simulink model "BMSOut"  (R2024a)
settings: Solver=FixedStepDiscrete  StartTime=0.0  StopTime=10000  RelTol=1e-3
undefined symbols (not defined in the file): PlntBattNumCellSer
settings Model: DataDictionary=VirtualVehicleTemplate.sldd  ModifiedByFormat=The MathWorks, Inc.  ExtModeTrigDuration=5  Creator=The MathWorks, Inc.  LastModifiedBy=The MathWorks, Inc.
settings SolverCC: AlgebraicLoopSolver=TrustRegion  PositivePriorityOrder=on  AutoInsertRateTranBlk=on  MaxZcPerStep=1
settings DataIOCC: ExternalInput=Battery  SaveOutput=off  SaveTime=off  SignalLoggingName=logsOut
settings OptimizationCC: BlockReduction=off  DefaultParameterBehavior=Inlined  UseFloatMulNetSlope=on  DefaultUnderspecifiedDataType=single  OptimizeBlockIOStorage=off  EnhancedBackFolding=on  PassReuseOutputArgsThreshold=0  ZeroExternalMemoryAtStartup=off  ZeroInternalMemoryAtStartup=off  EfficientFloat2IntCast=on  MaxStackSize=64  OptimizeBlockOrder=speed  DifferentSizesBufferReuse=on
settings DebuggingCC: SignalInfNanChecking=error  SaveWithParameterizedLinksMsg=none  CheckExecutionContextPreStartOutputMsg=on  IntegerOverflowMsg=error  ParameterPrecisionLossMsg=none  ParameterTunabilityLossMsg=error  UnconnectedInputMsg=warning  UnconnectedOutputMsg=warning  UnconnectedLineMsg=warning  AssertControl=DisableAll  PregeneratedLibrarySubsystemCodeDiagnostic=none  SFUnexpectedBacktrackingDiag=warning  SFNoUnconditionalDefaultTransitionDiag=warning  SFExecutionAtInitializationDiag=none  ArithmeticOperatorsInVariantConditions=warning
settings HardwareCC: ProdBitPerLong=64  ProdLongLongMode=on  ProdHWDeviceType=Intel->x86-64 (Linux 64)
settings ModelReferenceCC: EnableRefExpFcnMdlSchedulingChecks=on  ModelReferenceNumInstancesAllowed=Single  PropagateSignalLabelsOutOfModel=off
settings SFSimCC: SimUseLocalCustomCode=off  MATLABDynamicMemAlloc=off  CustomCodeUndefinedFunction=UseInterfaceOnly
settings RTWCC: GenerateReport=on  RTWUseLocalCustomCode=off  Toolchain=Simulink Real-Time Toolchain  BuildConfiguration=Faster Runs  TargetLang=C++  GPUComputeCapability=3.5  DLArmComputeVersion=19.05
settings CodeAppCC: ForceParamTrailComments=on  MaxIdLength=51  OperatorAnnotations=on  MangleLength=4
settings GRTTargetCC: TargetLangStandard=C++03 (ISO)  CodeInterfacePackaging=C++ class
settings ConfigComp: CovMetricSettings=dcw  CovSaveCumulativeToWorkspaceVar=on  CovSaveSingleToWorkspaceVar=on  CovExternalEMLEnable=off  CovSFcnEnable=off  DVMode=DesignErrorDetection  DVMaxProcessTime=7000  DVTestSuiteOptimization=Auto  DVDetectDeadLogic=on  DVDetectIntegerOverflow=off  DVRebuildModelRepresentation=Always

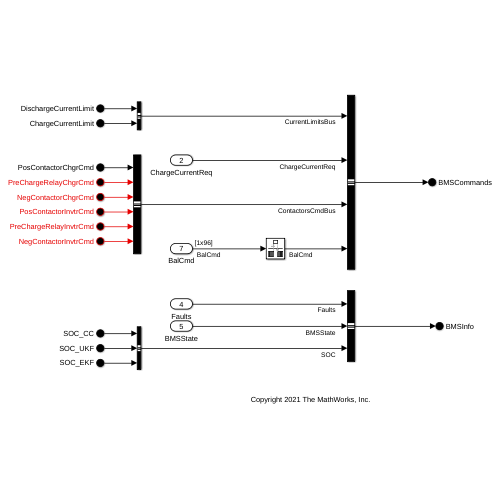
[thumbnail: Simulink's stored preview of the top-level diagram]
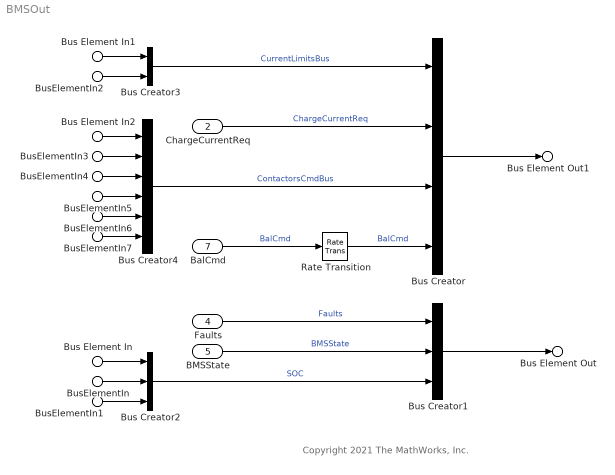
== system BMSOut ==
  note: Copyright 2021 The MathWorks, Inc.
  Bus Element In1 : Inport  PortName=CurrentLimits  Element=DischargeCurrentLimit
  BusElementIn2 : Inport  PortName=CurrentLimits  Element=ChargeCurrentLimit
  ChargeCurrentReq : Inport  Port=2  OutDataTypeStr=single  PortDimensions=1  SampleTime=[0.10000000000000001,0]
  Bus Element In2 : Inport  Port=3  PortName=Contactors_Cmd  Element=PosContactorChgrCmd
  BusElementIn3 : Inport  Port=3  PortName=Contactors_Cmd  Element=PreChargeRelayChgrCmd
  BusElementIn4 : Inport  Port=3  PortName=Contactors_Cmd  Element=NegContactorChgrCmd
  BusElementIn5 : Inport  Port=3  PortName=Contactors_Cmd  Element=PosContactorInvtrCmd
  BusElementIn6 : Inport  Port=3  PortName=Contactors_Cmd  Element=PreChargeRelayInvtrCmd
  BusElementIn7 : Inport  Port=3  PortName=Contactors_Cmd  Element=NegContactorInvtrCmd
  Faults : Inport  Port=4  OutDataTypeStr=boolean
  BMSState : Inport  Port=5  PortDimensions=1  SampleTime=[0.10000000000000001,0]
  Bus Element In : Inport  Port=6  PortName=SOC  Element=SOC_CC
  BusElementIn : Inport  Port=6  PortName=SOC  Element=SOC_UKF
  BusElementIn1 : Inport  Port=6  PortName=SOC  Element=SOC_EKF
  BalCmd : Inport  Port=7  OutDataTypeStr=boolean  PortDimensions=[1 PlntBattNumCellSer]  SampleTime=[5,0]
  Bus Creator1 : BusCreator  Inputs=3
  Bus Creator2 : BusCreator  Inputs=3
  Bus Creator3 : BusCreator  Inputs=2
  Bus Creator4 : BusCreator  Inputs=6
  Bus Creator : BusCreator  Inputs=4
  Rate Transition : RateTransition  Integrity=off  Deterministic=off
  Bus Element Out1 : Outport  PortName=BMSCommands
  Bus Element Out : Outport  Port=2  PortName=BMSInfo
  wires:
  Bus Creator1/1 -> Bus Element Out/1
  BusElementIn4/1 -> Bus Creator4/3
  Bus Element In2/1 -> Bus Creator4/1
  BusElementIn2/1 -> Bus Creator3/2
  BusElementIn3/1 -> Bus Creator4/2
  BusElementIn/1 -> Bus Creator2/2
  Bus Creator/1 -> Bus Element Out1/1
  BusElementIn6/1 -> Bus Creator4/5
  Bus Creator4/1 -> Bus Creator/3  "ContactorsCmdBus"
  BusElementIn1/1 -> Bus Creator2/3
  ChargeCurrentReq/1 -> Bus Creator/2  "ChargeCurrentReq"
  BusElementIn7/1 -> Bus Creator4/6
  Rate Transition/1 -> Bus Creator/4  "BalCmd"
  BusElementIn5/1 -> Bus Creator4/4
  Bus Creator2/1 -> Bus Creator1/3  "SOC"
  BalCmd/1 -> Rate Transition/1  "BalCmd"
  BMSState/1 -> Bus Creator1/2  "BMSState"
  Faults/1 -> Bus Creator1/1  "Faults"
  Bus Creator3/1 -> Bus Creator/1  "CurrentLimitsBus"
  Bus Element In/1 -> Bus Creator2/1
  Bus Element In1/1 -> Bus Creator3/1
